simulink model "controller"  (Simulink 7.7)
settings: Solver=FixedStepDiscrete  StartTime=0.0  StopTime=inf  RelTol=1e-3
InitFcn:
  | initRov14;
values from neighbouring files (symbols this model uses):
  k = [ 20   5   15 ... (first row only)    [initRov14.m]    (also in initSharedMem.m = [ 0*20   0*5   0*15)
  kw = 1    [initSharedMem.m]
  nc = 12    [initSharedMem.m]
  nj = 25    [initSharedMem.m]
undefined symbols (not defined in the file or in its folder): DiscIntNeverNeededParam
libraries: WBCLibrary x16, simulink x3, dspsigops x3
settings Model: Creator=daniele  LastModifiedBy=iron
settings DataIOCC: SignalLoggingSaveFormat=Dataset
settings DebuggingCC: FcnCallInpInsideContextMsg=Enable All

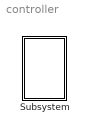
== system controller ==
  Subsystem : Subsystem  mask{robotName='icubGazeboSim', Ts=0.01, localName='dynamicBalancing'}
      mask prompts: robotName "robot name"; localName "module name"

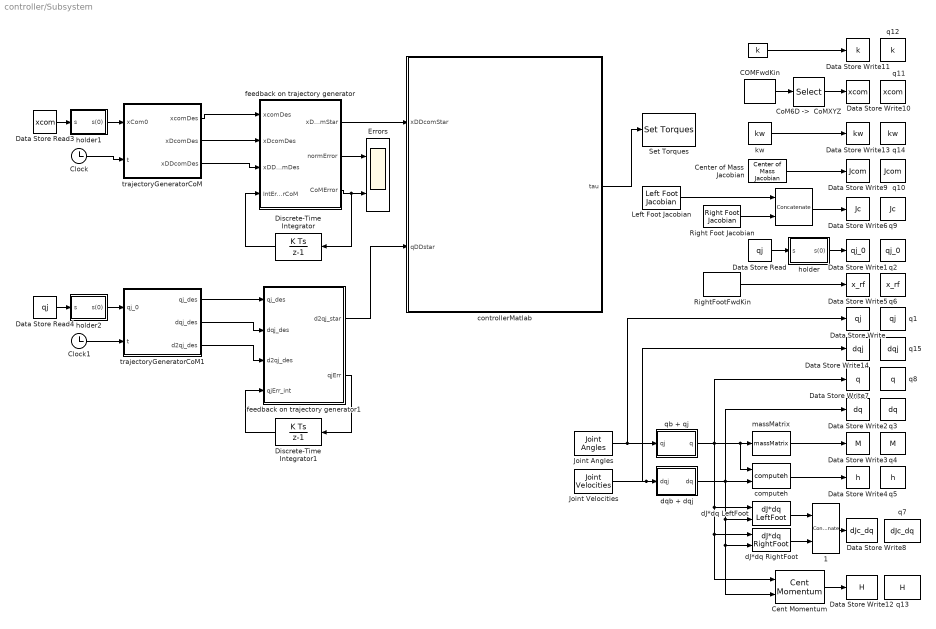
== system controller/Subsystem ==
  "    " : Constant  Value=k
  " " : Concatenate  Mode=Multidimensional array
  " 1" : Concatenate  Mode=Multidimensional array
  "COMFwdKin " : WBCLibrary/wholeBodyModel/Forward Kinematics/COMFwdKin   SystemSampleTime=-1  robotName=robotName  localName=localName
  Cent Momentum : WBCLibrary/wholeBodyModel/Dynamics/Cent Momentum  SystemSampleTime=-1  robotName=robotName  localName=localName
  Center of Mass Jacobian : WBCLibrary/wholeBodyModel/Jacobians/Center of Mass Jacobian  SystemSampleTime=-1  robotName=robotName  localName=localName
  Clock : Clock
      settings: Decimation=10
  Clock1 : Clock
      settings: Decimation=10
  "CoM6D ->  CoMXYZ" : Selector  InputPortWidth=7  IndexOptions=Index vector (dialog)  Indices=[1 2 3]  OutputSizes=1
  Data Store Read : DataStoreRead  DataStoreName=qj
  Data Store Read3 : DataStoreRead  DataStoreName=xcom
  Data Store Read4 : DataStoreRead  DataStoreName=qj
  Data Store Write : DataStoreWrite  DataStoreName=qj
  Data Store Write1 : DataStoreWrite  DataStoreName=qj_0
  Data Store Write10 : DataStoreWrite  DataStoreName=xcom
  Data Store Write11 : DataStoreWrite  DataStoreName=k
  Data Store Write12 : DataStoreWrite  DataStoreName=H
  Data Store Write13 : DataStoreWrite  DataStoreName=kw
  Data Store Write14 : DataStoreWrite  DataStoreName=dqj
  Data Store Write2 : DataStoreWrite  DataStoreName=dq
  Data Store Write3 : DataStoreWrite  DataStoreName=M
  Data Store Write4 : DataStoreWrite  DataStoreName=h
  Data Store Write5 : DataStoreWrite  DataStoreName=x_rf
  Data Store Write6 : DataStoreWrite  DataStoreName=Jc
  Data Store Write7 : DataStoreWrite  DataStoreName=q
  Data Store Write8 : DataStoreWrite  DataStoreName=dJc_dq
  Data Store Write9 : DataStoreWrite  DataStoreName=Jcom
  Discrete-Time Integrator : DiscreteIntegrator  InitialCondition=[0;0;0]  SampleTime=Ts  ICPrevOutput=DiscIntNeverNeededParam  ICPrevScaledInput=DiscIntNeverNeededParam
  Discrete-Time Integrator1 : DiscreteIntegrator  InitialCondition=zeros(nj,1)  SampleTime=Ts  ICPrevOutput=DiscIntNeverNeededParam  ICPrevScaledInput=DiscIntNeverNeededParam
  Errors : Scope  NumInputPorts=2
      settings: TimeRange=70  YMin=0~-0.045  YMax=0.0475~0.05  SaveName=ScopeData6
  Joint Angles : WBCLibrary/wholeBodyStates/Joint Angles  SystemSampleTime=-1  robotName=robotName  localName=localName
  Joint Velocities : WBCLibrary/wholeBodyStates/Joint Velocities  SystemSampleTime=-1  robotName=robotName  localName=localName
  Left Foot Jacobian : WBCLibrary/wholeBodyModel/Jacobians/Left Foot Jacobian  SystemSampleTime=-1  robotName=robotName  localName=localName
  Right Foot Jacobian : WBCLibrary/wholeBodyModel/Jacobians/Right Foot Jacobian  SystemSampleTime=-1  robotName=robotName  localName=localName
  RightFootFwdKin : WBCLibrary/wholeBodyModel/Forward Kinematics/RightFootFwdKin  SystemSampleTime=-1  robotName=robotName  localName=localName
  Set Torques : WBCLibrary/wholeBodyActuators/Set Torques  SystemSampleTime=-1  val=6  robotName=robotName  localName=localName
  computeh : WBCLibrary/wholeBodyModel/Dynamics/computeh  SystemSampleTime=-1  val=7  robotname=robotName  localname=localName
  controllerMatlab : Stateflow chart  TreatAsAtomicUnit=on
  dJ*dq LeftFoot : WBCLibrary/wholeBodyModel/Dynamics/dJ*dq LeftFoot  SystemSampleTime=-1  val=9  robotName=robotName  localName=localName
  dJ*dq RightFoot : WBCLibrary/wholeBodyModel/Dynamics/dJ*dq RightFoot  SystemSampleTime=-1  val=9  robotName=robotName  localName=localName
  dqb + dqj : Subsystem
  feedback on trajectory generator : Stateflow chart  TreatAsAtomicUnit=on
  feedback on trajectory generator1 : Stateflow chart  TreatAsAtomicUnit=on
  holder : Subsystem
  holder1 : Subsystem
  holder2 : Subsystem
  kw : Constant  Value=kw
  massMatrix : WBCLibrary/wholeBodyModel/Dynamics/massMatrix  SystemSampleTime=-1  val=8  robotname=robotName  localname=localName
  q1 : DataStoreMemory  DataStoreName=qj  ReadBeforeWriteMsg=warning  WriteAfterWriteMsg=warning  WriteAfterReadMsg=warning  InitialValue=zeros(nj,1)  VectorParams1D=off  OutDataTypeStr=double
  q10 : DataStoreMemory  DataStoreName=Jcom  ReadBeforeWriteMsg=warning  WriteAfterWriteMsg=warning  WriteAfterReadMsg=warning  InitialValue=zeros(6,nj+6)  VectorParams1D=off  OutDataTypeStr=double
  q11 : DataStoreMemory  DataStoreName=xcom  ReadBeforeWriteMsg=warning  WriteAfterWriteMsg=warning  WriteAfterReadMsg=warning  InitialValue=zeros(3,1)  VectorParams1D=off  OutDataTypeStr=double
  q12 : DataStoreMemory  DataStoreName=k  ReadBeforeWriteMsg=warning  WriteAfterWriteMsg=warning  WriteAfterReadMsg=warning  InitialValue=k  VectorParams1D=off  OutDataTypeStr=double
  q13 : DataStoreMemory  DataStoreName=H  ReadBeforeWriteMsg=warning  WriteAfterWriteMsg=warning  WriteAfterReadMsg=warning  InitialValue=zeros(6,1)  VectorParams1D=off  OutDataTypeStr=double
  q14 : DataStoreMemory  DataStoreName=kw  ReadBeforeWriteMsg=warning  WriteAfterWriteMsg=warning  WriteAfterReadMsg=warning  InitialValue=kw  VectorParams1D=off  OutDataTypeStr=double
  q15 : DataStoreMemory  DataStoreName=dqj  ReadBeforeWriteMsg=warning  WriteAfterWriteMsg=warning  WriteAfterReadMsg=warning  InitialValue=zeros(nj,1)  VectorParams1D=off  OutDataTypeStr=double
  q2 : DataStoreMemory  DataStoreName=qj_0  ReadBeforeWriteMsg=warning  WriteAfterWriteMsg=warning  WriteAfterReadMsg=warning  InitialValue=zeros(nj,1)  VectorParams1D=off  OutDataTypeStr=double
  q3 : DataStoreMemory  DataStoreName=dq  ReadBeforeWriteMsg=warning  WriteAfterWriteMsg=warning  WriteAfterReadMsg=warning  InitialValue=zeros(nj+6,1)  VectorParams1D=off  OutDataTypeStr=double
  q4 : DataStoreMemory  DataStoreName=M  ReadBeforeWriteMsg=warning  WriteAfterWriteMsg=warning  WriteAfterReadMsg=warning  InitialValue=zeros(nj+6,nj+6)  VectorParams1D=off  OutDataTypeStr=double
  q5 : DataStoreMemory  DataStoreName=h  ReadBeforeWriteMsg=warning  WriteAfterWriteMsg=warning  WriteAfterReadMsg=warning  InitialValue=zeros(nj+6,1)  VectorParams1D=off  OutDataTypeStr=double
  q6 : DataStoreMemory  DataStoreName=x_rf  ReadBeforeWriteMsg=warning  WriteAfterWriteMsg=warning  WriteAfterReadMsg=warning  InitialValue=zeros(7,1)  VectorParams1D=off  OutDataTypeStr=double
  q7 : DataStoreMemory  DataStoreName=dJc_dq  ReadBeforeWriteMsg=warning  WriteAfterWriteMsg=warning  WriteAfterReadMsg=warning  InitialValue=zeros(nc,1)  VectorParams1D=off  OutDataTypeStr=double
  q8 : DataStoreMemory  DataStoreName=q  ReadBeforeWriteMsg=warning  WriteAfterWriteMsg=warning  WriteAfterReadMsg=warning  InitialValue=zeros(nj+16,1)  VectorParams1D=off  OutDataTypeStr=double
  q9 : DataStoreMemory  DataStoreName=Jc  ReadBeforeWriteMsg=warning  WriteAfterWriteMsg=warning  WriteAfterReadMsg=warning  InitialValue=zeros(nc,nj+6)  VectorParams1D=off  OutDataTypeStr=double
  qb + qj : Subsystem
  trajectoryGeneratorCoM : Stateflow chart  TreatAsAtomicUnit=on
  trajectoryGeneratorCoM1 : Stateflow chart  TreatAsAtomicUnit=on
  wires:
  Left Foot Jacobian/1 -> " "/1
  Right Foot Jacobian/1 -> " "/2
  qb + qj/1(q) -> Data Store Write7/1, massMatrix/1, computeh/1, dJ*dq LeftFoot/1, Cent Momentum/1, dJ*dq RightFoot/1
  dqb + dqj/1(dq) -> computeh/2, Data Store Write2/1, dJ*dq LeftFoot/2, Cent Momentum/2, dJ*dq RightFoot/2
  Data Store Read/1 -> holder/1(s)
  holder/1(s(0)) -> Data Store Write1/1
  massMatrix/1 -> Data Store Write3/1
  computeh/1 -> Data Store Write4/1
  Joint Velocities/1 -> dqb + dqj/1(dqj), Data Store Write14/1
  RightFootFwdKin/1 -> Data Store Write5/1
  " "/1 -> Data Store Write6/1
  "    "/1 -> Data Store Write11/1
  Center of Mass Jacobian/1 -> Data Store Write9/1
  "COMFwdKin "/1 -> "CoM6D ->  CoMXYZ"/1
  "CoM6D ->  CoMXYZ"/1 -> Data Store Write10/1
  Clock/1 -> trajectoryGeneratorCoM/2(t)
  holder1/1(s(0)) -> trajectoryGeneratorCoM/1(xCom0)
  dJ*dq LeftFoot/1 -> " 1"/1
  dJ*dq RightFoot/1 -> " 1"/2
  " 1"/1 -> Data Store Write8/1
  Cent Momentum/1 -> Data Store Write12/1
  kw/1 -> Data Store Write13/1
  controllerMatlab/1(tau) -> Set Torques/1
  Data Store Read3/1 -> holder1/1(s)
  trajectoryGeneratorCoM/1(xcomDes) -> feedback on trajectory generator/1(xcomDes)
  trajectoryGeneratorCoM/2(xDcomDes) -> feedback on trajectory generator/2(xDcomDes)
  trajectoryGeneratorCoM/3(xDDcomDes) -> feedback on trajectory generator/3(xDDcomDes)
  feedback on trajectory generator/1(xDDcomStar) -> controllerMatlab/1(xDDcomStar)
  Discrete-Time Integrator/1 -> feedback on trajectory generator/4(IntErrorCoM)
  feedback on trajectory generator/2(normError) -> Errors/1
  Clock1/1 -> trajectoryGeneratorCoM1/2(t)
  holder2/1(s(0)) -> trajectoryGeneratorCoM1/1(qj_0)
  Data Store Read4/1 -> holder2/1(s)
  trajectoryGeneratorCoM1/1(qj_des) -> feedback on trajectory generator1/1(qj_des)
  trajectoryGeneratorCoM1/2(dqj_des) -> feedback on trajectory generator1/2(dqj_des)
  trajectoryGeneratorCoM1/3(d2qj_des) -> feedback on trajectory generator1/3(d2qj_des)
  Discrete-Time Integrator1/1 -> feedback on trajectory generator1/4(qjErr_int)
  feedback on trajectory generator1/2(qjErr) -> Discrete-Time Integrator1/1
  Joint Angles/1 -> qb + qj/1(qj), Data Store Write/1
  feedback on trajectory generator/3(CoMError) -> Errors/2, Discrete-Time Integrator/1
  feedback on trajectory generator1/1(d2qj_star) -> controllerMatlab/2(qDDstar)

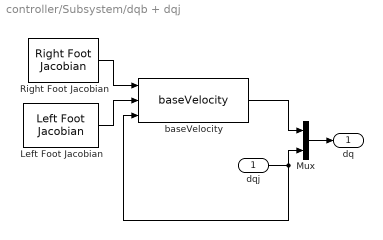
== system controller/Subsystem/dqb + dqj ==
  dqj : Inport
  Left Foot Jacobian : WBCLibrary/wholeBodyModel/Jacobians/Left Foot Jacobian  SystemSampleTime=-1  robotName=robotName  localName=localName
  Mux : Mux  Inputs=2
  Right Foot Jacobian : WBCLibrary/wholeBodyModel/Jacobians/Right Foot Jacobian  SystemSampleTime=-1  robotName=robotName  localName=localName
  baseVelocity : WBCLibrary/Utilities/baseVelocity  SystemSampleTime=-1
  dq : Outport
  wires:
  Left Foot Jacobian/1 -> baseVelocity/2
  Right Foot Jacobian/1 -> baseVelocity/1
  baseVelocity/1 -> Mux/1
  dqj/1 -> baseVelocity/3, Mux/2
  Mux/1 -> dq/1

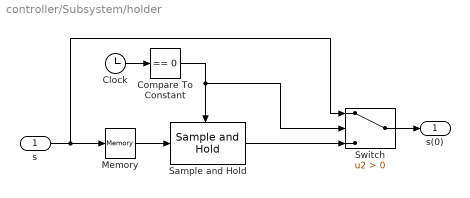
== system controller/Subsystem/holder ==
  s : Inport
  Clock : Clock
      settings: Decimation=10
  Compare To Constant : simulink/Logic and Bit Operations/Compare To Constant  SystemSampleTime=-1  relop===  const=0  LogicOutDataTypeMode=boolean
  Memory : Memory
  Sample and Hold : dspsigops/Sample and Hold  SystemSampleTime=-1  trig=Falling edge  initCond=0  latchinput=off
  Switch : Switch  Criteria=u2 > Threshold
  s(0) : Outport
  wires:
  s/1 -> Switch/1, Memory/1
  Clock/1 -> Compare To Constant/1
  Compare To Constant/1 -> Sample and Hold/Trigger, Switch/2
  Sample and Hold/1 -> Switch/3
  Switch/1 -> s(0)/1
  Memory/1 -> Sample and Hold/1

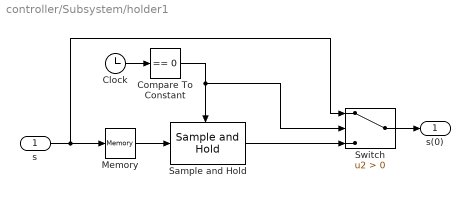
== system controller/Subsystem/holder1 ==
  s : Inport
  Clock : Clock
      settings: Decimation=10
  Compare To Constant : simulink/Logic and Bit Operations/Compare To Constant  SystemSampleTime=-1  relop===  const=0  LogicOutDataTypeMode=boolean
  Memory : Memory
  Sample and Hold : dspsigops/Sample and Hold  SystemSampleTime=-1  trig=Falling edge  initCond=0  latchinput=off
  Switch : Switch  Criteria=u2 > Threshold
  s(0) : Outport
  wires:
  s/1 -> Switch/1, Memory/1
  Clock/1 -> Compare To Constant/1
  Compare To Constant/1 -> Sample and Hold/Trigger, Switch/2
  Sample and Hold/1 -> Switch/3
  Switch/1 -> s(0)/1
  Memory/1 -> Sample and Hold/1

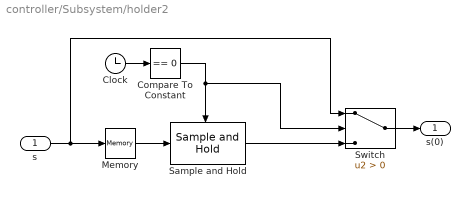
== system controller/Subsystem/holder2 ==
  s : Inport
  Clock : Clock
      settings: Decimation=10
  Compare To Constant : simulink/Logic and Bit Operations/Compare To Constant  SystemSampleTime=-1  relop===  const=0  LogicOutDataTypeMode=boolean
  Memory : Memory
  Sample and Hold : dspsigops/Sample and Hold  SystemSampleTime=-1  trig=Falling edge  initCond=0  latchinput=off
  Switch : Switch  Criteria=u2 > Threshold
  s(0) : Outport
  wires:
  s/1 -> Switch/1, Memory/1
  Clock/1 -> Compare To Constant/1
  Compare To Constant/1 -> Sample and Hold/Trigger, Switch/2
  Sample and Hold/1 -> Switch/3
  Switch/1 -> s(0)/1
  Memory/1 -> Sample and Hold/1

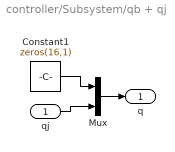
== system controller/Subsystem/qb + qj ==
  qj : Inport
  Constant1 : Constant  Value=zeros(16,1)
  Mux : Mux  Inputs=2
  q : Outport
  wires:
  Mux/1 -> q/1
  Constant1/1 -> Mux/1
  qj/1 -> Mux/2

== matlab function Subsystem/trajectoryGeneratorCoM ==
  data: xcomDes output double; xCom0 input double; t input double; Jcom data_store_memory double; xDcomDes output double; xDDcomDes output double; dq data_store_memory double; k data_store_memory double
function [xcomDes, xDcomDes, xDDcomDes]  = trajGen(xCom0,t)
%#codegen


e3 = [0;1;0];
A = 0.1;
f = 0.1;
t = t*0.8;
% xcomDes    = [xCom0(1:2); (1/A-1)*A*xCom0(3)] + A*xCom0(3)*cos(2*pi*f*t)*e3;
% xDcomDes   = -xCom0(3)*A*2*pi*f*sin(2*pi*f*t)*e3;
% xDDcomDes  = -xCom0(3)*A*(2*pi*f)^2*cos(2*pi*f*t)*e3;

xcomDes    = xCom0 + A*sin(2*pi*f*t)*e3;
xDcomDes   =         A*2*pi*f*cos(2*pi*f*t)*e3;
xDDcomDes  =        -A*(2*pi*f)^2*sin(2*pi*f*t)*e3;

== matlab function Subsystem/controllerMatlab ==
  data: qj data_store_memory double; qj_0 data_store_memory double; dq data_store_memory double; M data_store_memory double; h data_store_memory double; x_rf data_store_memory double; Jc data_store_memory double; tau output double; xcom data_store_memory double; xDDcomStar input double; H data_store_memory double; dJc_dq data_store_memory double; k data_store_memory double; kw data_store_memory double; qDDstar input double
function tau  = computeTau(xDDcomStar, qDDstar)
%#codegen

global qj dq qj_0 
global M h Jc dJc_dq H
global x_rf xcom k kw

nt = 25;

PINV_TOL = 1e-5;
g        = 9.81;

DL = 25-nt;            %DeltaIndexOnlyLegs

if DL ~= 0
   Jcr = [Jc(:,1:6),Jc(:,7 + DL:end)]; 
else
   Jcr = Jc; 
end

m     = M(1,1);
Mb    = M(1:6,1:6);
MbInv = inv(Mb);
Mbj   = M(1:6,7 + DL :end); 
Mj    = M(7 + DL :end,7 + DL:end);
U     = [eye(6) , zeros(6,nt)];
Jcb   = Jcr*U';
SBar  = [  -MbInv*Mbj 
           eye(nt)      ];
NjInv = Mj - Mbj'*MbInv*Mbj;

grav = [zeros(2,1);-m*g;zeros(3,1)];

JcSBar     = Jcr*SBar;
JcSBarPinv = pinv(JcSBar, PINV_TOL);

% Definition of reference accelerations for CoM and Joints that ensure
% stabilization of desired trajectories xDcomDes and qDes 

if DL ~= 0
   q_star = qDDstar(DL+1:end); 
else
   q_star = qDDstar;
    
end
Pr =  x_rf(1:3) - xcom; % Application point of the contact force on the right foot w.r.t. CoM
A  = [ eye(3),   zeros(3),eye(3), zeros(3);
      -Sf(xcom),  eye(3), Sf(Pr), eye(3) ];

% The following expressions for Ic and IcD hold only if the control 
% objective is the stabilization of the CoM's position
% kw = 0.1;
hwDotDes = H(4:end);
hDotDes = [ m*xDDcomStar ;
            -kw*hwDotDes  ]; 

fd = pinv(A)*(hDotDes-grav);

LambdaStar = JcSBarPinv*(Jcb*MbInv*(h(1:6) - Jcb'*fd) - dJc_dq);

NP0 = eye(nt) - JcSBarPinv*JcSBar;

LambdaStar = LambdaStar + NP0 * q_star;

tauLegs = - JcSBar'*fd + NjInv*LambdaStar + SBar'*[h(1:6);h(DL + 7:end)];

if DL ~= 0
   tau = h(7:end) - k(3,1)*(qj - qj_0) - k(3,3)*dq(7:end);   
   tau(DL+1:end) = tauLegs;
else
    tau = tauLegs;
end

== matlab function Subsystem/feedback on trajectory generator ==
  data: xDDcomStar output double; normError output double; xcomDes input double; xDcomDes input double; xDDcomDes input double; IntErrorCoM input double; Jcom data_store_memory double; CoMError output double; dq data_store_memory double; k data_store_memory double; xcom data_store_memory double
function [xDDcomStar, normError, CoMError]  = fcn(xcomDes, xDcomDes, xDDcomDes, IntErrorCoM)
%#codegen

global Jcom dq k xcom

xDcom      = Jcom(1:3,:)*dq;
xDDcomStar = xDDcomDes - k(1,1)*(xcom - xcomDes) - k(1,2)*IntErrorCoM - k(1,3)*(xDcom - xDcomDes)  ;

CoMError    = xcom - xcomDes;
normError   = norm(CoMError);

== matlab function Subsystem/feedback on trajectory generator1 ==
  data: d2qj_star output double; qj_des input double; dqj_des input double; d2qj_des input double; qjErr output double; Jcom data_store_memory double; k data_store_memory double; qjErr_int input double; qj data_store_memory double; dqj data_store_memory double
function [d2qj_star, qjErr]   = fcn(qj_des, dqj_des, d2qj_des, qjErr_int)
%#codegen

global k qj dqj

d2qj_star   = d2qj_des - k(2,1)*(qj - qj_des) - k(2,2)*qjErr_int- k(2,3)*(dqj - dqj_des);

qjErr = qj - qj_des;

== matlab function Subsystem/trajectoryGeneratorCoM1 ==
  data: qj_des output double; qj_0 input double; t input double; Jcom data_store_memory double; dqj_des output double; d2qj_des output double; dq data_store_memory double; k data_store_memory double
function [qj_des, dqj_des, d2qj_des]  = trajGen(qj_0,t)
%#codegen


qj_des    = qj_0;
dqj_des   = zeros(size(qj_0));
d2qj_des  = zeros(size(qj_0));
